simulink model "iter_imas_contr_4"  (Simulink 8.5)
settings: Solver=ode1  StartTime=EqTime  StopTime=1e8  FixedStep=SimStep  MaxStep=5.e-3  MinStep=2e-4  RelTol=1.e-3
undefined symbols (not defined in the file): Elong, g1, g1_term, g2, g2_term, g3, g3_term, g4, g4_term, g5, g5_term, g6, g6_term, Imax, key_imas, n_gaps, n_mc, ncam, npf, ntur, RupRd, scr_data, SimStep, Vcspf_up, vec_imas, volt
libraries: simulink x56
(part 3 of 3)

== system iter_imas_contr_4/kavin_contr/Control1/controllers/Lim. contr.1/gain_cont2 ==
  Time : Inport
  Data Store Read : DataStoreRead  DataStoreName=tcont2  DataStoreElements=tcont2
  Data Store Read1 : DataStoreRead  DataStoreName=dtcont2  DataStoreElements=dtcont2
  Divide2 : Product  Inputs=*/
  Saturation1 : Saturate  UpperLimit=1  LowerLimit=0
  Subtract3 : Sum  Inputs=+-
  Out1 : Outport
  wires:
  Data Store Read/1 -> Subtract3/2
  Time/1 -> Subtract3/1
  Subtract3/1 -> Divide2/1
  Data Store Read1/1 -> Divide2/2
  Divide2/1 -> Saturation1/1
  Saturation1/1 -> Out1/1

== system iter_imas_contr_4/kavin_contr/Control1/controllers/Lim. contr.1/t_cont2 ==
  errlim : Inport
  Time : Inport  Port=2
  Data Store Read : DataStoreRead  DataStoreName=tcont2  DataStoreElements=tcont2
  Divide12 : Product  Inputs=**
  Relational Operator : RelationalOperator  Operator=>  OutDataTypeStr=float('double')
  Out1 : Outport
  wires:
  errlim/1 -> Divide12/1
  Time/1 -> Relational Operator/1
  Data Store Read/1 -> Relational Operator/2
  Relational Operator/1 -> Divide12/2
  Divide12/1 -> Out1/1

== system iter_imas_contr_4/kavin_contr/Control1/controllers/Lim. contr.1/t_cont2_1 ==
  lim. contr. : Inport
  Time : Inport  Port=2
  Curr. cont. : Inport  Port=3
  " 1 " : Switch  Threshold=1
  1 : Switch  Threshold=1
  Data Store Read : DataStoreRead  DataStoreName=tcont2  DataStoreElements=tcont2
  Data Store Read1 : DataStoreRead  DataStoreName=tdiv  DataStoreElements=tdiv
  Memory2 : Memory
  Relational Operator : RelationalOperator  Operator=>  OutDataTypeStr=float('double')
  Relational Operator1 : RelationalOperator  OutDataTypeStr=float('double')
  Out1 : Outport
  wires:
  Time/1 -> Relational Operator1/1, Relational Operator/1
  Data Store Read/1 -> Relational Operator/2
  Relational Operator/1 -> 1/2
  lim. contr./1 -> 1/1
  Curr. cont./1 -> 1/3
  " 1 "/1 -> Memory2/1, Out1/1
  1/1 -> " 1 "/3
  Memory2/1 -> " 1 "/1
  Data Store Read1/1 -> Relational Operator1/2
  Relational Operator1/1 -> " 1 "/2

== system iter_imas_contr_4/kavin_contr/Control1/controllers/curr term contr/Curr. term. contr ==
  In1 : Inport
  S-Function : S-Function  FunctionName=contr_curr  Parameters=20,n_mc,2  SFunctionModules='contr_curr_wrapper'
  Selector : Selector  InputPortWidth=20  Indices=[1:n_mc]
  Out1 : Outport
  wires:
  Selector/1 -> Out1/1
  In1/1 -> S-Function/1
  S-Function/1 -> Selector/1

== system iter_imas_contr_4/kavin_contr/Control1/controllers/curr term contr/term tr ==
  Time : Inport
  Data Store Read2 : DataStoreRead  DataStoreName=tterm
  Relational Operator2 : RelationalOperator  OutDataTypeStr=float('double')
  Out1 : Outport
  wires:
  Time/1 -> Relational Operator2/1
  Data Store Read2/1 -> Relational Operator2/2
  Relational Operator2/1 -> Out1/1

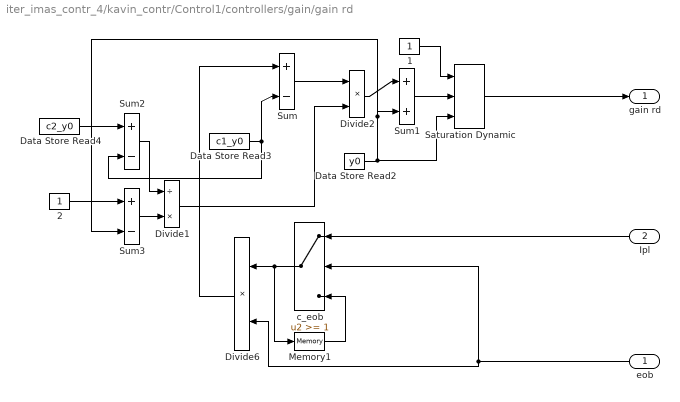
== system iter_imas_contr_4/kavin_contr/Control1/controllers/gain/gain rd ==
  eob : Inport
  Ipl : Inport  Port=2
  1 : Constant
  2 : Constant
  Data Store Read2 : DataStoreRead  DataStoreName=y0  DataStoreElements=y0
  Data Store Read3 : DataStoreRead  DataStoreName=c1_y0  DataStoreElements=c1_y0
  Data Store Read4 : DataStoreRead  DataStoreName=c2_y0  DataStoreElements=c2_y0
  Divide1 : Product  Inputs=/*
  Divide2 : Product  Inputs=**
  Divide6 : Product  Inputs=**
  Memory1 : Memory
  Saturation Dynamic : simulink/Discontinuities/Saturation Dynamic  OutMin=[]  OutMax=[]  OutDataTypeStr=Inherit: Same as second input  OutDataType=fixdt(1, 16)  OutScaling=2^-10  DoSatur=off
  Sum : Sum  Inputs=|+-
  Sum1 : Sum  Inputs=|++
  Sum2 : Sum  Inputs=+-
  Sum3 : Sum  Inputs=+-
  c_eob : Switch  Threshold=1
  gain rd : Outport
  wires:
  Data Store Read3/1 -> Sum2/2, Sum/2
  Data Store Read2/1 -> Saturation Dynamic/3, Sum3/2, Sum1/2
  Divide2/1 -> Sum1/1
  Sum/1 -> Divide2/1
  Divide6/1 -> Sum/1
  c_eob/1 -> Divide6/1, Memory1/1
  eob/1 -> Divide6/2, c_eob/2
  Memory1/1 -> c_eob/3
  Ipl/1 -> c_eob/1
  1/1 -> Saturation Dynamic/1
  Data Store Read4/1 -> Sum2/1
  2/1 -> Sum3/1
  Sum3/1 -> Divide1/2
  Sum2/1 -> Divide1/1
  Divide1/1 -> Divide2/2
  Sum1/1 -> Saturation Dynamic/2
  Saturation Dynamic/1 -> gain rd/1
